simulink model "Model_InterpretationEngine64"  (R2022b)
settings: Solver=FixedStepDiscrete  StartTime=0.0  StopTime=5  RelTol=1e-3  EnableMultiTasking=on
InitFcn:
  | % Initialize model
  | ModelSettings=BTConfig.GetModelSettings();
  | 
  | ModelSettings.Validate();
  | 
  | ModelInit;
  | 
  | 
  | % load library data
  | GainLibrary_data;
  | % Load saved values from partition process
  | CapturedConstMask.LoadMapFromFile(bdroot)
  | % Load saved values from partition process
  | TSP_Mask.LoadMapFromFile(bdroot)
StartFcn:
  | % make sure all the simulated RTC requests are found
  | %RTC_SIM_OBJ.ValidateREQs();
undefined symbols (not defined in the file or in its folder): NumHFRefBPF, NumHFRefLPF
libraries: StateVar x112, TSP x56, FeaturePath x24
(part 5 of 5)

== system Model_InterpretationEngine64/ModelPreAmp/DecRate/AudioPilot35/Audiopilot_3_5/NoiseEstimationVariant/RegularNoiseEstimation/LFNoiseEstimatorCoh/SpeedBoundsAndNoiseSlew/SpeedBounds ==
  "CurrentMaximum " : Subsystem  mask(Talaria Target State Variable){TriggerInit=[805 511 945 569], TspName=CurrMax, StateName=CurrMax, UseSameName=on, IfdefMacro=[]}
      mask prompts: TriggerInit "Hidden: MoveFcn redraw"; TspName "Name:"; StateName "Name of StateVar:"; UseSameName "Use same name for state variable and TSP"; IfdefMacro "Additional #ifdef macro to enable trigger capture:"
      mask help: The TargetStateVar block encapsultes a Target State Probe (TSP), a State Variable, and a Trivial Interpretation between them.
      mask init:
      | [ok,tspPath,activeStatePath] = TargetStateVarMask.Init(gcbh);
      settings: MoveFcn=TargetStateVarMask.CB_TriggerInit(gcbh);
      mask Help: See help for StateVar and TSP blocks
      mask Callback TriggerInit: TargetStateVarMask.CB_TriggerInit(gcbh);
      mask TypeOptions TspName: TSP/TspName
      mask TypeOptions StateName: StateVar/StateName
      mask Callback UseSameName: TargetStateVarMask.CB_UseSameName(gcbh);
      mask TypeOptions IfdefMacro: TSP/IfdefMacro
      mask DialogControl AdvancedPanel Prompt: Advanced
      mask DialogControl ConvertToFullInterpretation Prompt: Irreversible conversion to full interpretation
      mask DialogControl ConvertToFullInterpretation Callback: TargetStateVarMask.CB_ConvertToFullInterpretation(gcbh);
      mask DialogControl ErrorContainer Prompt: Error Messages
      mask DialogControl ErrorText Prompt: The interpreted StateVar value is not yet available
      mask DialogControl TspPathText Prompt: TSP: Current parameter name: [AudiopilotLfNoiseSpeedBoundsCurrMax]
      mask Display:
      | % retrieve icon definition
      | [path,w,h] = TargetStateVarMask.Icon();
      | 
      | % retrieve the block's pixel size
      | pos = get(gcbh,'position');
      | bw = pos(3) - pos(1);
      | bh = pos(4) - pos(2);
      | 
      | % draw centered icon
      | xAdj = bw/2 - w/2 + 5;
      | yAdj = bh/2 - h/2 + 4;
      | for i=1:length(path)
      | 	patch(path(i).x+xAdj, path(i).y+yAdj, path(i).rgb);
      | end
      | 
      | % show the top name or an X
      | if (exist('ok','var') && ok)
      | 	text(bw*0.5, bh*0.2, tspPath, 'horizontalAlignment', 'center');
      | 	patch(0,0,[1 1 1]);
      | 	patch(bw,bh,[1 1 1]);
      | else
      | 	tx=bw*0.03;
      | 	ty=bh*0.03;
      | 	patch([0 tx bw bw-tx], [ty 0 bh-ty bh], [1 0 0]);
      | 	patch([0 bw-tx bw tx], [bh-ty 0 ty bh], [1 0 0]);
      | end
  CurrentMinimum : Subsystem  mask(Talaria Target State Variable){TriggerInit=[805 431 945 489], TspName=CurrMin, StateName=CurrMin, UseSameName=on, IfdefMacro=[]}
      mask prompts: TriggerInit "Hidden: MoveFcn redraw"; TspName "Name:"; StateName "Name of StateVar:"; UseSameName "Use same name for state variable and TSP"; IfdefMacro "Additional #ifdef macro to enable trigger capture:"
      mask help: The TargetStateVar block encapsultes a Target State Probe (TSP), a State Variable, and a Trivial Interpretation between them.
      mask init:
      | [ok,tspPath,activeStatePath] = TargetStateVarMask.Init(gcbh);
      settings: MoveFcn=TargetStateVarMask.CB_TriggerInit(gcbh);
      mask Help: See help for StateVar and TSP blocks
      mask Callback TriggerInit: TargetStateVarMask.CB_TriggerInit(gcbh);
      mask TypeOptions TspName: TSP/TspName
      mask TypeOptions StateName: StateVar/StateName
      mask Callback UseSameName: TargetStateVarMask.CB_UseSameName(gcbh);
      mask TypeOptions IfdefMacro: TSP/IfdefMacro
      mask DialogControl AdvancedPanel Prompt: Advanced
      mask DialogControl ConvertToFullInterpretation Prompt: Irreversible conversion to full interpretation
      mask DialogControl ConvertToFullInterpretation Callback: TargetStateVarMask.CB_ConvertToFullInterpretation(gcbh);
      mask DialogControl ErrorContainer Prompt: Error Messages
      mask DialogControl ErrorText Prompt: The interpreted StateVar value is not yet available
      mask DialogControl TspPathText Prompt: TSP: Current parameter name: [AudiopilotLfNoiseSpeedBoundsCurrMin]
      mask Display:
      | % retrieve icon definition
      | [path,w,h] = TargetStateVarMask.Icon();
      | 
      | % retrieve the block's pixel size
      | pos = get(gcbh,'position');
      | bw = pos(3) - pos(1);
      | bh = pos(4) - pos(2);
      | 
      | % draw centered icon
      | xAdj = bw/2 - w/2 + 5;
      | yAdj = bh/2 - h/2 + 4;
      | for i=1:length(path)
      | 	patch(path(i).x+xAdj, path(i).y+yAdj, path(i).rgb);
      | end
      | 
      | % show the top name or an X
      | if (exist('ok','var') && ok)
      | 	text(bw*0.5, bh*0.2, tspPath, 'horizontalAlignment', 'center');
      | 	patch(0,0,[1 1 1]);
      | 	patch(bw,bh,[1 1 1]);
      | else
      | 	tx=bw*0.03;
      | 	ty=bh*0.03;
      | 	patch([0 tx bw bw-tx], [ty 0 bh-ty bh], [1 0 0]);
      | 	patch([0 bw-tx bw tx], [bh-ty 0 ty bh], [1 0 0]);
      | end
  FeaturePath : FeaturePath/FeaturePath  FeatureName=SpeedBounds  IsGroup=off  GroupNumber=-1  IsModule=off  TriggerInit=[115 194 230 301]
      settings: SourceProductName=Bose Talaria
  Flag : Subsystem  mask(Talaria Target State Variable){TriggerInit=[805 351 945 409], TspName=Flag, StateName=Flag, UseSameName=on, IfdefMacro=[]}
      mask prompts: TriggerInit "Hidden: MoveFcn redraw"; TspName "Name:"; StateName "Name of StateVar:"; UseSameName "Use same name for state variable and TSP"; IfdefMacro "Additional #ifdef macro to enable trigger capture:"
      mask help: The TargetStateVar block encapsultes a Target State Probe (TSP), a State Variable, and a Trivial Interpretation between them.
      mask init:
      | [ok,tspPath,activeStatePath] = TargetStateVarMask.Init(gcbh);
      settings: MoveFcn=TargetStateVarMask.CB_TriggerInit(gcbh);
      mask Help: See help for StateVar and TSP blocks
      mask Callback TriggerInit: TargetStateVarMask.CB_TriggerInit(gcbh);
      mask TypeOptions TspName: TSP/TspName
      mask TypeOptions StateName: StateVar/StateName
      mask Callback UseSameName: TargetStateVarMask.CB_UseSameName(gcbh);
      mask TypeOptions IfdefMacro: TSP/IfdefMacro
      mask DialogControl AdvancedPanel Prompt: Advanced
      mask DialogControl ConvertToFullInterpretation Prompt: Irreversible conversion to full interpretation
      mask DialogControl ConvertToFullInterpretation Callback: TargetStateVarMask.CB_ConvertToFullInterpretation(gcbh);
      mask DialogControl ErrorContainer Prompt: Error Messages
      mask DialogControl ErrorText Prompt: The interpreted StateVar value is not yet available
      mask DialogControl TspPathText Prompt: TSP: Current parameter name: [AudiopilotLfNoiseSpeedBoundsFlag]
      mask Display:
      | % retrieve icon definition
      | [path,w,h] = TargetStateVarMask.Icon();
      | 
      | % retrieve the block's pixel size
      | pos = get(gcbh,'position');
      | bw = pos(3) - pos(1);
      | bh = pos(4) - pos(2);
      | 
      | % draw centered icon
      | xAdj = bw/2 - w/2 + 5;
      | yAdj = bh/2 - h/2 + 4;
      | for i=1:length(path)
      | 	patch(path(i).x+xAdj, path(i).y+yAdj, path(i).rgb);
      | end
      | 
      | % show the top name or an X
      | if (exist('ok','var') && ok)
      | 	text(bw*0.5, bh*0.2, tspPath, 'horizontalAlignment', 'center');
      | 	patch(0,0,[1 1 1]);
      | 	patch(bw,bh,[1 1 1]);
      | else
      | 	tx=bw*0.03;
      | 	ty=bh*0.03;
      | 	patch([0 tx bw bw-tx], [ty 0 bh-ty bh], [1 0 0]);
      | 	patch([0 bw-tx bw tx], [bh-ty 0 ty bh], [1 0 0]);
      | end

== system Model_InterpretationEngine64/ModelPreAmp/DecRate/AudioPilot35/Audiopilot_3_5/NoiseEstimationVariant/RegularNoiseEstimation/HFNoiseEstimatorCoh/HfNoiseMusicSeparation /MicPsdLevel/TargetStateVar ==
  StateVar : StateVar/StateVar  TriggerInit=[490 139 605 201]  StateName=MicPsdLevel
      settings: SourceProductName=Bose Talaria
  TSP : TSP/TSP  TriggerInit=[110 134 215 206]  TspName=MicPsdLevel  IfDefMacro=IfdefMacro  Role=Automatic
      settings: SourceProductName=Bose Talaria
  TrivialInterpretation : StateVar/TrivialInterpretation  TriggerInit=[330 148 380 192]
      settings: SourceProductName=Bose Talaria
  wires:
  TSP/1 -> TrivialInterpretation/1
  TrivialInterpretation/1 -> StateVar/1

== system Model_InterpretationEngine64/ModelPreAmp/DecRate/AudioPilot35/Audiopilot_3_5/NoiseEstimationVariant/RegularNoiseEstimation/HFNoiseEstimatorCoh/PostProcessing/HfImpulseRejection/MinSearch ==
  Flatness : Subsystem  mask(Talaria Target State Variable){TriggerInit=[700 271 945 339], TspName=Flatness, StateName=Flatness, UseSameName=on, IfdefMacro=[]}
      mask prompts: TriggerInit "Hidden: MoveFcn redraw"; TspName "Name:"; StateName "Name of StateVar:"; UseSameName "Use same name for state variable and TSP"; IfdefMacro "Additional #ifdef macro to enable trigger capture:"
      mask help: The TargetStateVar block encapsultes a Target State Probe (TSP), a State Variable, and a Trivial Interpretation between them.
      mask init:
      | [ok,tspPath,activeStatePath] = TargetStateVarMask.Init(gcbh);
      settings: MoveFcn=TargetStateVarMask.CB_TriggerInit(gcbh);
      mask Help: See help for StateVar and TSP blocks
      mask Callback TriggerInit: TargetStateVarMask.CB_TriggerInit(gcbh);
      mask TypeOptions TspName: TSP/TspName
      mask TypeOptions StateName: StateVar/StateName
      mask Callback UseSameName: TargetStateVarMask.CB_UseSameName(gcbh);
      mask TypeOptions IfdefMacro: TSP/IfdefMacro
      mask DialogControl AdvancedPanel Prompt: Advanced
      mask DialogControl ConvertToFullInterpretation Prompt: Irreversible conversion to full interpretation
      mask DialogControl ConvertToFullInterpretation Callback: TargetStateVarMask.CB_ConvertToFullInterpretation(gcbh);
      mask DialogControl ErrorContainer Prompt: Error Messages
      mask Display:
      | % retrieve icon definition
      | [path,w,h] = TargetStateVarMask.Icon();
      | 
      | % retrieve the block's pixel size
      | pos = get(gcbh,'position');
      | bw = pos(3) - pos(1);
      | bh = pos(4) - pos(2);
      | 
      | % draw centered icon
      | xAdj = bw/2 - w/2 + 5;
      | yAdj = bh/2 - h/2 + 4;
      | for i=1:length(path)
      | 	patch(path(i).x+xAdj, path(i).y+yAdj, path(i).rgb);
      | end
      | 
      | % show the top name or an X
      | if (exist('ok','var') && ok)
      | 	text(bw*0.5, bh*0.2, tspPath, 'horizontalAlignment', 'center');
      | 	patch(0,0,[1 1 1]);
      | 	patch(bw,bh,[1 1 1]);
      | else
      | 	tx=bw*0.03;
      | 	ty=bh*0.03;
      | 	patch([0 tx bw bw-tx], [ty 0 bh-ty bh], [1 0 0]);
      | 	patch([0 bw-tx bw tx], [bh-ty 0 ty bh], [1 0 0]);
      | end

== system Model_InterpretationEngine64/ModelPreAmp/DecRate/AudioPilot35/Audiopilot_3_5/NoiseEstimationVariant/RegularNoiseEstimation/HFNoiseEstimatorCoh/PostProcessing/HfImpulseRejection/Pmin ==
  StateVar : StateVar/StateVar  TriggerInit=[490 139 605 201]  StateName=Pmin
      settings: SourceProductName=Bose Talaria
  TSP : TSP/TSP  TriggerInit=[110 134 215 206]  TspName=Pmin  IfDefMacro=IfdefMacro  Role=Automatic
      settings: SourceProductName=Bose Talaria
  TrivialInterpretation : StateVar/TrivialInterpretation  TriggerInit=[330 148 380 192]
      settings: SourceProductName=Bose Talaria
  wires:
  TSP/1 -> TrivialInterpretation/1
  TrivialInterpretation/1 -> StateVar/1

== system Model_InterpretationEngine64/ModelPreAmp/DecRate/AudioPilot35/Audiopilot_3_5/NoiseEstimationVariant/RegularNoiseEstimation/LFNoiseEstimatorCoh/SpeedBoundsAndNoiseSlew/SpeedBounds/CurrentMaximum  ==
  StateVar : StateVar/StateVar  TriggerInit=[490 139 605 201]  StateName=CurrMax
      settings: SourceProductName=Bose Talaria
  TSP : TSP/TSP  TriggerInit=[110 134 215 206]  TspName=CurrMax  IfDefMacro=IfdefMacro  Role=Automatic
      settings: SourceProductName=Bose Talaria
  TrivialInterpretation : StateVar/TrivialInterpretation  TriggerInit=[330 148 380 192]
      settings: SourceProductName=Bose Talaria
  wires:
  TSP/1 -> TrivialInterpretation/1
  TrivialInterpretation/1 -> StateVar/1

== system Model_InterpretationEngine64/ModelPreAmp/DecRate/AudioPilot35/Audiopilot_3_5/NoiseEstimationVariant/RegularNoiseEstimation/LFNoiseEstimatorCoh/SpeedBoundsAndNoiseSlew/SpeedBounds/CurrentMinimum ==
  StateVar : StateVar/StateVar  TriggerInit=[490 139 605 201]  StateName=CurrMin
      settings: SourceProductName=Bose Talaria
  TSP : TSP/TSP  TriggerInit=[110 134 215 206]  TspName=CurrMin  IfDefMacro=IfdefMacro  Role=Automatic
      settings: SourceProductName=Bose Talaria
  TrivialInterpretation : StateVar/TrivialInterpretation  TriggerInit=[330 148 380 192]
      settings: SourceProductName=Bose Talaria
  wires:
  TSP/1 -> TrivialInterpretation/1
  TrivialInterpretation/1 -> StateVar/1

== system Model_InterpretationEngine64/ModelPreAmp/DecRate/AudioPilot35/Audiopilot_3_5/NoiseEstimationVariant/RegularNoiseEstimation/LFNoiseEstimatorCoh/SpeedBoundsAndNoiseSlew/SpeedBounds/Flag ==
  StateVar : StateVar/StateVar  TriggerInit=[490 139 605 201]  StateName=Flag
      settings: SourceProductName=Bose Talaria
  TSP : TSP/TSP  TriggerInit=[110 134 215 206]  TspName=Flag  IfDefMacro=IfdefMacro  Role=Automatic
      settings: SourceProductName=Bose Talaria
  TrivialInterpretation : StateVar/TrivialInterpretation  TriggerInit=[330 148 380 192]
      settings: SourceProductName=Bose Talaria
  wires:
  TSP/1 -> TrivialInterpretation/1
  TrivialInterpretation/1 -> StateVar/1

== system Model_InterpretationEngine64/ModelPreAmp/DecRate/AudioPilot35/Audiopilot_3_5/NoiseEstimationVariant/RegularNoiseEstimation/HFNoiseEstimatorCoh/PostProcessing/HfImpulseRejection/MinSearch/Flatness ==
  StateVar : StateVar/StateVar  TriggerInit=[490 139 605 201]  StateName=Flatness
      settings: SourceProductName=Bose Talaria
  TSP : TSP/TSP  TriggerInit=[110 134 215 206]  TspName=Flatness  IfDefMacro=IfdefMacro  Role=Automatic
      settings: SourceProductName=Bose Talaria
  TrivialInterpretation : StateVar/TrivialInterpretation  TriggerInit=[330 148 380 192]
      settings: SourceProductName=Bose Talaria
  wires:
  TSP/1 -> TrivialInterpretation/1
  TrivialInterpretation/1 -> StateVar/1

== matlab function Model_InterpretationEngine64/ModelPreAmp/DecRate/AudioPilot35/Audiopilot_3_5/NoiseEstimationVariant/RegularNoiseEstimation/LFNoiseEstimatorCoh/LfNoiseImpulseRejection/ImpulseVariance/db20 ==
  data: State output; TSP1 input
  events: trigger input FUNCTION_CALL_EVENT
function State  = fcn(TSP1)
%#codegen

State = db20(abs(TSP1)+eps);

== matlab function Model_InterpretationEngine64/ModelPreAmp/DecRate/AudioPilot35/Audiopilot_3_5/NoiseEstimationVariant/RegularNoiseEstimation/HFNoiseEstimatorCoh/HfNoiseMusicSeparation /NoisePsdLevel/ExtractNoiseLevel ==
  data: PSD input; NoiseLevel output
  events: trigger input FUNCTION_CALL_EVENT
function NoiseLevel  = fcn(PSD)
% This sums the Power Spectral Density values across all
% frequency bands.
%#codegen

NoiseLevel = sum(PSD);

== matlab function Model_InterpretationEngine64/ModelPreAmp/DecRate/AudioPilot35/Audiopilot_3_5/NoiseEstimationVariant/RegularNoiseEstimation/LFNoiseEstimatorCoh/LfNoiseImpulseRejection/GammaTauS/GammaConversion ==
  data: State output; Coef input; DecRate3 parameter
  events: trigger input FUNCTION_CALL_EVENT
function State  = fcn(Coef,DecRate3)
% Converts the filter coefficient back to time constant
%#codegen

% Keep all values single
one1 = single(1.0);
zero1 = single(0.0);

% Handle the divide-by-zero case
if (Coef == one1)
    State = zero1;
else
    State = one1 / ((one1 - Coef)*DecRate3);
end

== matlab function Model_InterpretationEngine64/ModelPreAmp/DecRate/AudioPilot35/Audiopilot_3_5/NoiseEstimationVariant/RegularNoiseEstimation/LFNoiseEstimatorCoh/LfNoiseImpulseRejection/MusicVariance/db20  ==
  data: State output; TSP1 input
  events: trigger input FUNCTION_CALL_EVENT
function State  = fcn(TSP1)
%#codegen

State = db20(abs(TSP1) + eps);

== matlab function Model_InterpretationEngine64/ModelPreAmp/DecRate/AudioPilot35/Audiopilot_3_5/NoiseEstimationVariant/RegularNoiseEstimation/LFNoiseEstimatorCoh/LfNoiseImpulseRejection/NoiseVariance/db20  ==
  data: State output; TSP1 input
  events: trigger input FUNCTION_CALL_EVENT
function State  = fcn(TSP1)
%#codegen

State = db20(abs(TSP1) + eps);

== matlab function Model_InterpretationEngine64/ModelPreAmp/DecRate/AudioPilot35/Audiopilot_3_5/NoiseEstimationVariant/RegularNoiseEstimation/LFNoiseEstimatorCoh/LfNoiseImpulseRejection/TotalVariance/db20  ==
  data: State output; TSP1 input
  events: trigger input FUNCTION_CALL_EVENT
function State  = fcn(TSP1)
%#codegen

State = db20(abs(TSP1) + eps);
